simulink model "secon_example1"  (Simulink 8.7)
settings: Solver=ode45  StartTime=0.0  StopTime=100  RelTol=1e-3
libraries: simulink x1, fuzblock x1
settings Model: Creator=home2  LastModifiedBy=mohamed
settings DataIOCC: SignalLoggingSaveFormat=ModelDataLogs
settings DebuggingCC: SolverPrmCheckMsg=warning  FcnCallInpInsideContextMsg=UseLocalSettings  StateNameClashWarn=warning
settings GRTTargetCC: CombineOutputUpdateFcns=off  GRTInterface=on

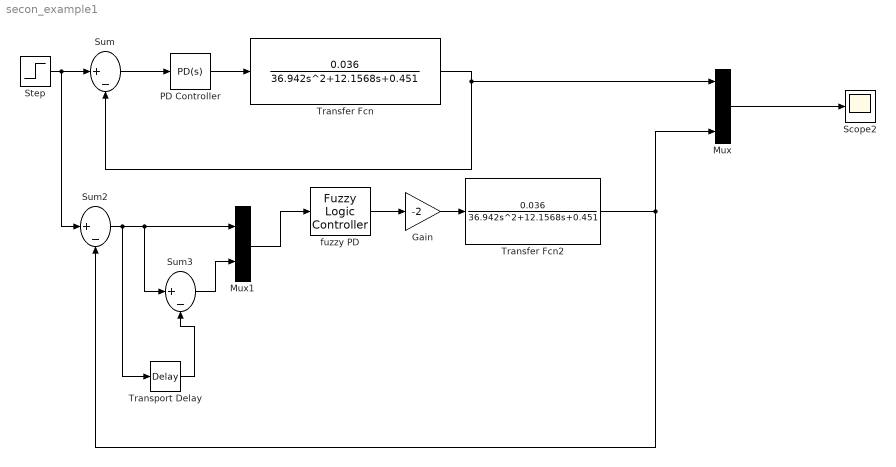
== system secon_example1 ==
  Gain : Gain  Gain=-2
  Mux : Mux  Inputs=3
  Mux1 : Mux  Inputs=2
  PD Controller : simulink/Continuous/PID Controller  Controller=PD  TimeDomain=Continuous-time  SampleTime=-1  IntegratorMethod=Forward Euler  FilterMethod=Forward Euler  Form=Parallel  UseFilter=on  ControllerParametersSource=internal  P=99  I=1  D=1  N=30  InitialConditionSource=internal  InitialConditionForIntegrator=0  InitialConditionForFilter=0  ExternalReset=none  LimitOutput=off  UpperSaturationLimit=inf  LowerSaturationLimit=-inf  LinearizeAsGain=on  AntiWindupMode=none  Kb=1  TrackingMode=off  Kt=1  PParamMin=[]  PParamMax=[]  IParamMin=[]  IParamMax=[]  DParamMin=[]  DParamMax=[]  NParamMin=[]  NParamMax=[]  KbParamMin=[]  KbParamMax=[]  KtParamMin=[]  KtParamMax=[]  POutMin=[]  POutMax=[]  IOutMin=[]  IOutMax=[]  DOutMin=[]  DOutMax=[]  NOutMin=[]  NOutMax=[]  KbOutMin=[]  KbOutMax=[]  KtOutMin=[]  KtOutMax=[]  IntegratorOutMin=[]  IntegratorOutMax=[]  FilterOutMin=[]  FilterOutMax=[]  SumOutMin=[]  SumOutMax=[]  SumI1OutMin=[]  SumI1OutMax=[]  SumI2OutMin=[]  SumI2OutMax=[]  SumI3OutMin=[]  SumI3OutMax=[]  SumDOutMin=[]  SumDOutMax=[]  SaturationOutMin=[]  SaturationOutMax=[]  IntegratorContinuousStateAttributes=''  IntegratorStateMustResolveToSignalObject=off  IntegratorRTWStateStorageClass=Auto  FilterContinuousStateAttributes=''  FilterStateMustResolveToSignalObject=off  FilterRTWStateStorageClass=Auto  DifferentiatorICPrevScaledInput=0  DifferentiatorOutMin=[]  DifferentiatorOutMax=[]
  Scope2 : Scope
  Step : Step  Time=0  SampleTime=0
  Sum : Sum  Inputs=|+-
  Sum2 : Sum  Inputs=|+-
  Sum3 : Sum  Inputs=|+-
  Transfer Fcn : TransferFcn  Numerator=[0.036]  Denominator=[36.942 12.1568 0.451]
  Transfer Fcn2 : TransferFcn  Numerator=[0.036]  Denominator=[36.942 12.1568 0.451]
  Transport Delay : TransportDelay
  fuzzy PD : fuzblock/Fuzzy Logic  Controller  fis=ex2
  wires:
  PD Controller/1 -> Transfer Fcn/1
  Transfer Fcn/1 -> Sum/2, Mux/1
  Sum/1 -> PD Controller/1
  Mux/1 -> Scope2/1
  Transfer Fcn2/1 -> Sum2/2, Mux/3
  Step/1 -> Sum2/1, Sum/1
  Transport Delay/1 -> Sum3/2
  Sum3/1 -> Mux1/2
  Mux1/1 -> fuzzy PD/1
  Sum2/1 -> Transport Delay/1, Mux1/1, Sum3/1
  Gain/1 -> Transfer Fcn2/1
  fuzzy PD/1 -> Gain/1
